simulink model "ROS2Simulink"  (R2023b)
settings: Solver=VariableStepAuto  StartTime=0.0  StopTime=inf  RelTol=1e-3
undefined symbols (not defined in the file or in its folder): Angular, Linear
libraries: robotlib x2
settings Model: Creator=Renzhaofu  LastModifiedBy=Renzhaofu

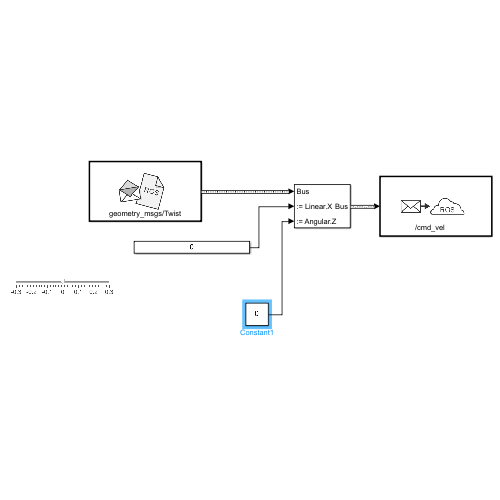
[thumbnail: Simulink's stored preview of the top-level diagram]
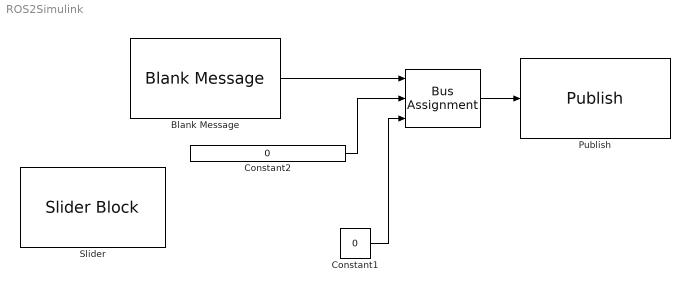
== system ROS2Simulink ==
  " " : BusAssignment  AssignedSignals=Linear.X,Angular.Z
  Blank Message : robotlib/Blank Message  messageClass=Message  entityType=geometry_msgs/Twist  messageType=geometry_msgs/Twist  SampleTime=inf  legacyBusStruct=off
  Constant1 : Constant  Value=0
  Constant2 : Constant  Value=0
  Publish : robotlib/Publish  topicSource=Select from ROS network  topic=/cmd_vel  messageType=geometry_msgs/Twist  legacyBusStruct=off  messageQueueLength=1
  Slider : SliderBlock  LabelPosition=Hide  ScaleMin=-0.3  ScaleMax=+0.3
  wires:
  Blank Message/1 -> " "/1
  " "/1 -> Publish/1
  Constant1/1 -> " "/3
  Constant2/1 -> " "/2
